simulink model "qaff1"  (Simulink 3.00)
settings: Solver=ode45  SolverMode=SingleTasking  StartTime=0.0  StopTime=20  MaxStep=.010  RelTol=1e-3  AbsTol=1e-3
undefined symbols (not defined in the file or in its folder): at, bt, ct, dt
settings Model: TimeSaveName=t  SaveOutput=off

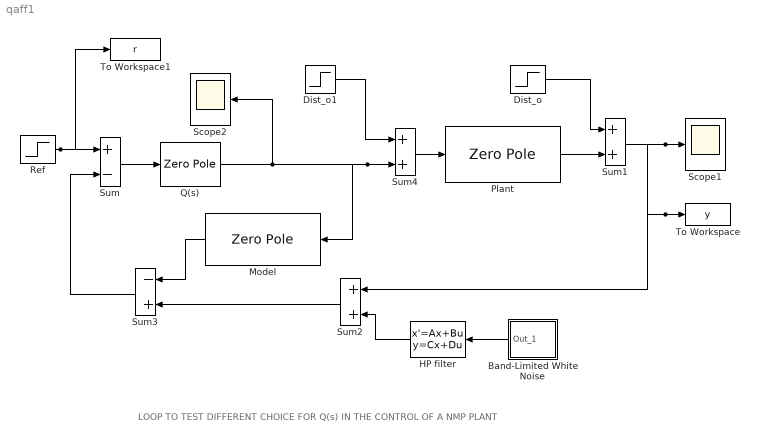
== system qaff1 ==
  note: LOOP TO TEST DIFFERENT CHOICE FOR Q(s) IN THE CONTROL OF A NMP PLANT
  Band-Limited White Noise : Subsystem  Orientation=left  mask(Continuous White Noise.){@1=[0.1], @2=0.1, @3=[23341]}
      mask prompts: @1 "Noise Power:"; @2 "Sample Time:"; @3 "Seed"
      mask help:
      | White noise for continuous (s-domain) systems.
      | Band-limited using zero-order-hold.
      mask init:
      | Cov = @1; Ts = @2; seed = @3; r = rand(1,12); r2 = [r(1),r;r,r(12)]; t =[1:13;1:13];
      mask Help: Implemented using white noise into Zero-Order Hold block. The seed and power can be vectors of the same length to produce a vector of white noise sources. For faster simulation, set sample time to the highest value possible but in accordance with the fastest dynamics of system.
      mask Display: plot(t(:),r2(:))
  Dist_o : Step  Time=10  Before=0  After=1  SampleTime=0
  Dist_o1 : Step  Time=10  Before=0  After=1  SampleTime=0
  HP filter : StateSpace  Orientation=left  A=at  B=bt  C=ct  D=dt  X0=0  mask(buttap,lp2hp){@1=0.5, @2=5}
      mask prompts: @1 "Cutoff frequency (rad/sec):"; @2 "Order"
      mask help:
      | Analog Butterworth high pass filter.
      |
      | (Requires Signal Processing Toolbox)
      mask init:
      | [at,bt,ct,dt,w,mag]=filtm('buttap','lp2hp',@1,[],20,@2);
      mask Help: Butterworth high pass filter using MATLAB's butter and lp2hp commands.
      mask Display: plot(w,mag)
  Model : ZeroPole  Orientation=left  Zeros=[2]  Poles=[-2; -1]  Gain=[-1]
  Plant : ZeroPole  Zeros=[2]  Poles=[-2; -1]  Gain=[-1]
  Q(s) : ZeroPole  Zeros=z  Poles=p  Gain=k  mask(buttap){@1=5, @2=4}
      mask prompts: @1 "Cutoff frequency (rad/sec)"; @2 "Order"
      mask help:
      | Analog Butterworth low pass filter.
      |
      | (Requires Signal Processing Toolbox)
      mask init:
      | [z,p,k]=buttap(@2); z=@1*z; p=@1*p; k=real(prod(-p)); [num,den]=zp2tf(z,p,k); w=logspace(log10(@1/10),log10(10*@1),20); h=freqs(num,den,w);
      mask Help: Butterworth low pass filter using MATLAB's butter command.
      mask Display: plot(20*log10(w),20*log10(abs(h)))
  Ref : Step  Time=1  Before=0  After=1  SampleTime=0
  Scope1 : Scope
      settings: TickLabels=on  TimeRange=20.000000  YMin=-2  YMax=2  SaveToWorkspace=off  SaveName=ScopeData  DataFormat=Matrix
  Scope2 : Scope
      settings: TickLabels=on  TimeRange=20.000000  YMin=-2.000000  YMax=2.000000  SaveToWorkspace=off  SaveName=ScopeData  DataFormat=Matrix
  Sum : Sum  Inputs=+-  SaturateOnIntegerOverflow=on
  Sum1 : Sum  Inputs=++  SaturateOnIntegerOverflow=on
  Sum2 : Sum  Orientation=left  Inputs=++  SaturateOnIntegerOverflow=on
  Sum3 : Sum  Orientation=left  Inputs=-+  SaturateOnIntegerOverflow=on
  Sum4 : Sum  Inputs=++  SaturateOnIntegerOverflow=on
  To Workspace : ToWorkspace  VariableName=y  SampleTime=0  SaveFormat=Matrix
      settings: Buffer=10000
  To Workspace1 : ToWorkspace  VariableName=r  SampleTime=0  SaveFormat=Matrix
      settings: Buffer=10000
  wires:
  Sum/1 -> Q(s)/1
  Dist_o/1 -> Sum1/1
  HP filter/1 -> Sum2/2
  Q(s)/1 -> Scope2/1, Sum4/2, Model/1
  Sum2/1 -> Sum3/2
  Model/1 -> Sum3/1
  Sum3/1 -> Sum/2
  Sum1/1 -> Scope1/1, Sum2/1, To Workspace/1
  Band-Limited White Noise/1(Out_1) -> HP filter/1
  Plant/1 -> Sum1/2
  Sum4/1 -> Plant/1
  Ref/1 -> Sum/1, To Workspace1/1
  Dist_o1/1 -> Sum4/1

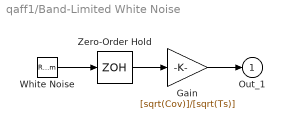
== system qaff1/Band-Limited White Noise ==
  Gain : Gain  Gain=[sqrt(Cov)]/[sqrt(Ts)]  SaturateOnIntegerOverflow=on
  White Noise : RandomNumber  Mean=0  Variance=1  Seed=seed  SampleTime=0
  Zero-Order Hold : ZeroOrderHold  SampleTime=Ts
  Out_1 : Outport  Port=1  InitialOutput=0
  wires:
  White Noise/1 -> Zero-Order Hold/1
  Gain/1 -> Out_1/1
  Zero-Order Hold/1 -> Gain/1
